simulink model "UnitTest_largeAttitude"  (R2020a)
settings: Solver=FixedStepAuto  StartTime=0.0  StopTime=511.0  FixedStep=0.01  RelTol=1e-3
settings Model: EnablePacing=on  PacingRate=3  Creator=Administrator  LastModifiedBy=Administrator

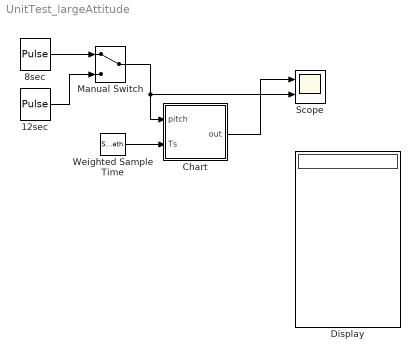
== system UnitTest_largeAttitude ==
  12sec : DiscretePulseGenerator  PulseType=Time based  Amplitude=60*pi/180  Period=3
  8sec : DiscretePulseGenerator  PulseType=Time based  Amplitude=60*pi/180  Period=30
  Chart : Stateflow chart  TreatAsAtomicUnit=on
  Display : Display
  Manual Switch : ManualSwitch
  Scope : Scope  NumInputPorts=2
  Weighted Sample Time : SampleTimeMath  TsampMathOp=Ts Only
  wires:
  Manual Switch/1 -> Scope/2, Chart/1(pitch)
  Weighted Sample Time/1 -> Chart/2(Ts)
  Chart/1(out) -> Scope/1
  8sec/1 -> Manual Switch/1
  12sec/1 -> Manual Switch/2
  ? -> Display/1

== stateflow chart UnitTest_largeAttitude/Chart ==
  state Work
    state normal
      en:
    state abnormal
      en:
    (default) -> normal
    normal -> abnormal : [isLargeAttitudeLong(pitch)]
    abnormal -> normal : [~isLargeAttitudeLong(pitch)]
  (default) -> Work
  data: flag_out function_output; pitch_in function_input; pitch input; Ts input; out output; flag_toAbnormal local
  function flag_out  = isLargeAttitudeLong(pitch_in):
    | function flag_out  = isLargeAttitudeLong(pitch_in)
    | persistent du period pitchFlagSet rollSet 
    | nFlag = 6;
    | if isempty(du)
    |     du = 0; 
    |     period = 0;
    |     pitchFlagSet = zeros(nFlag,1);
    | end
    | period = period + Ts;
    | threshold_pitch = 50*pi/180;
    | value_period = 5; % sec
    | if period >= value_period
    |     period = 0;
    |     pitchFlagSet(1:end-1) = pitchFlagSet(2:end);
    |     pitchFlagSet(end) = 0;
    | else
    |     % 在周期内，更新flag值
    |     if abs(pitch_in) > threshold_pitch
    |         pitchFlagSet(end) = 1;
    |     end
    | end
    | % if PathModeOut.flightTaskMode == ENUM_FlightTaskMode.GroundStandByMode 
    | 
    | %%
    | flag_out = false;
    | if sum(pitchFlagSet) > 2
    |     flag_out = true;
    | else
    |     flag_out = false;
    | end
    | % for i = 1:nFlag
    | %     pitchFlagSet_out(i) = pitchFlagSet(i);
    | % end
